simulink model "lead_compensation"  (R2018a)
settings: Solver=ode45  StartTime=0.0  StopTime=10.0  RelTol=1e-3  EnableMultiTasking=on
values from neighbouring files (symbols this model uses):
  K = 8    [params.m]
  Kt = 0.5    [params.m]
settings Model: ExtModeTrigMode=oneshot  ExtModeArmWhenConnect=off  Creator=eechris  LastModifiedBy=eechris
settings DataIOCC: SaveFormat=Array  SignalLoggingSaveFormat=ModelDataLogs
settings OptimizationCC: BlockReduction=off  BooleanDataType=off  ExpressionDepthLimit=2147483647  LifeSpan=inf
settings DebuggingCC: SaveWithParameterizedLinksMsg=none  UnderspecifiedInitializationDetection=Classic  MergeDetectMultiDrivingBlocksExec=none  SignalResolutionControl=TryResolveAllWithWarning  MultiTaskDSMMsg=warning  MultiTaskCondExecSysMsg=none  FcnCallInpInsideContextMsg=warning  StateNameClashWarn=warning  SFUnexpectedBacktrackingDiag=warning  SFNoUnconditionalDefaultTransitionDiag=warning  SFExecutionAtInitializationDiag=none
settings HardwareCC: ProdBitPerPointer=32  ProdBitPerSizeT=32  ProdBitPerPtrDiffT=32  ProdLargestAtomicFloat=None  ProdIntDivRoundTo=Undefined  ProdEndianess=Unspecified  ProdWordSize=32  ProdHWDeviceType=32-bit Generic  TargetUnknown=on
settings ModelReferenceCC: PropagateSignalLabelsOutOfModel=off
settings CodeAppCC: StateflowObjectComments=on
settings GRTTargetCC: TargetLangStandard=C89/C90 (ANSI)  GeneratePreprocessorConditionals=Disable all  CombineOutputUpdateFcns=off  GRTInterface=on
settings ConfigComp: CovMetricSettings=dw  CovHtmlReporting=on  CovSaveCumulativeToWorkspaceVar=on  CovSaveSingleToWorkspaceVar=on  CovExternalEMLEnable=off

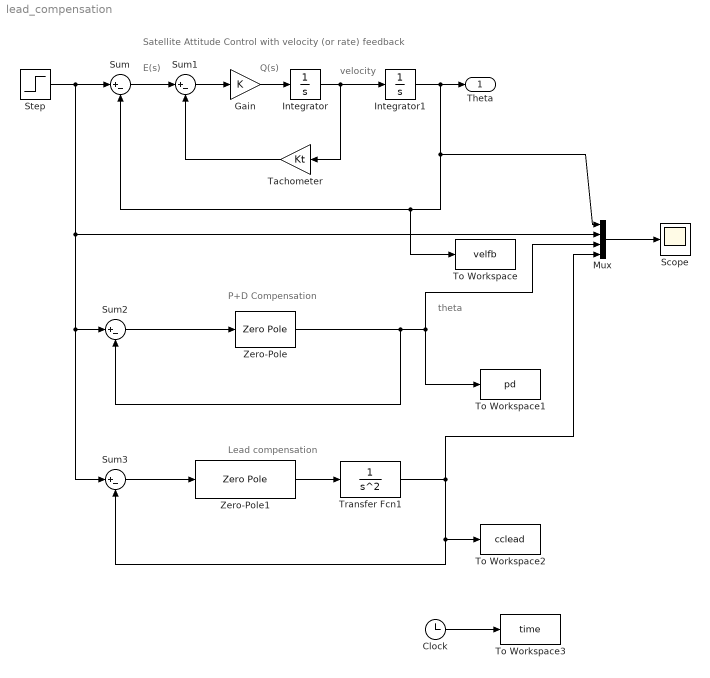
== system lead_compensation ==
  note: Satellite Attitude Control with velocity (or rate) feedback
  note: E(s)
  note: Q(s)
  note: velocity
  note: P+D Compensation
  note: theta
  note: Lead compensation
  Clock : Clock
  Gain : Gain  Gain=K  SaturateOnIntegerOverflow=on  OutDataTypeStr=Inherit: Same as input  ParamDataTypeStr=Inherit: Same as input
  Integrator : Integrator
  Integrator1 : Integrator
  Mux : Mux
  Scope : Scope
  Step : Step  Time=0  SampleTime=0
  Sum{,1..3} (4 alike) : Sum  Inputs=|+-  SaturateOnIntegerOverflow=on  InputSameDT=on  OutDataTypeStr=Inherit: Same as first input
  Tachometer : Gain  Gain=Kt  SaturateOnIntegerOverflow=on  OutDataTypeStr=Inherit: Same as input  ParamDataTypeStr=Inherit: Same as input
  To Workspace : ToWorkspace  VariableName=velfb  SampleTime=-1
  To Workspace1 : ToWorkspace  VariableName=pd  SampleTime=-1
  To Workspace2 : ToWorkspace  VariableName=cclead  SampleTime=-1
  To Workspace3 : ToWorkspace  VariableName=time  SampleTime=-1
  Transfer Fcn1 : TransferFcn  Denominator=[1 0 0]
  Zero-Pole : ZeroPole  Zeros=[-2]  Poles=[0, 0]  Gain=[K*Kt]
  Zero-Pole1 : ZeroPole  Zeros=[-1.1716]  Poles=[-6.8284 ]  Gain=[19.3137 ]
  Theta : Outport
  wires:
  Gain/1 -> Integrator/1
  Sum1/1 -> Gain/1
  Step/1 -> Sum/1, Mux/2, Sum2/1, Sum3/1
  Sum/1 -> Sum1/1
  Integrator/1 -> Integrator1/1, Tachometer/1
  Tachometer/1 -> Sum1/2
  Integrator1/1 -> Theta/1, Sum/2, To Workspace/1, Mux/1
  Sum2/1 -> Zero-Pole/1
  Zero-Pole/1 -> Sum2/2, To Workspace1/1, Mux/3
  Transfer Fcn1/1 -> Sum3/2, To Workspace2/1, Mux/4
  Zero-Pole1/1 -> Transfer Fcn1/1
  Sum3/1 -> Zero-Pole1/1
  Clock/1 -> To Workspace3/1
  Mux/1 -> Scope/1
